simulink model "ukol2"  (R2024b)
settings: Solver=VariableStepAuto  StartTime=0.0  StopTime=40000  RelTol=1e-3
settings Model: Creator=jirka  LastModifiedBy=jirka

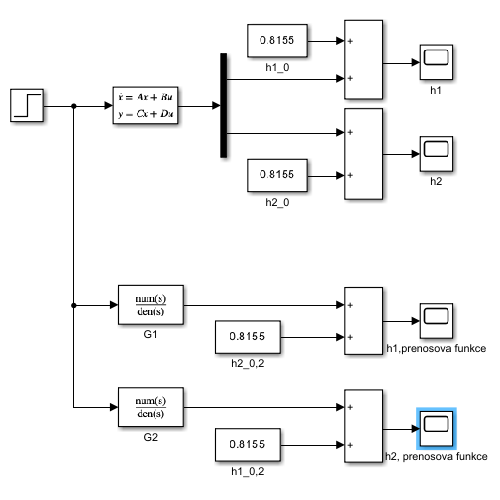
[thumbnail: Simulink's stored preview of the top-level diagram]
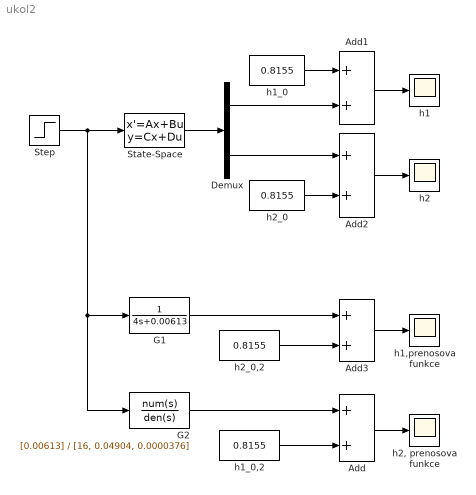
== system ukol2 ==
  Add{,1..3} (4 alike) : Sum
  Demux : Demux  Outputs=2
  G1 : TransferFcn  Denominator=[4, 0.00613]
  G2 : TransferFcn  Numerator=[0.00613]  Denominator=[16, 0.04904, 0.0000376]
  State-Space : StateSpace  A=[-0.00153 0; 0.00153 -0.00153]  B=[0.25; 0]  C=[1 0; 0 1]  D=[0; 0]  InitialCondition=0
  Step : Step  Time=20000  After=0.001  SampleTime=0
  h1 : Scope
  h1,prenosova funkce : Scope
  h1_0 : Constant  Value=0.8155
  h1_0,2 : Constant  Value=0.8155
  h2 : Scope
  "h2, prenosova funkce" : Scope
  h2_0 : Constant  Value=0.8155
  h2_0,2 : Constant  Value=0.8155
  wires:
  Step/1 -> G2/1, G1/1, State-Space/1
  State-Space/1 -> Demux/1
  Demux/2 -> Add2/1
  h1_0/1 -> Add1/1
  h2_0/1 -> Add2/2
  Add1/1 -> h1/1
  Add2/1 -> h2/1
  Demux/1 -> Add1/2
  G2/1 -> Add/1
  h1_0,2/1 -> Add/2
  Add/1 -> "h2, prenosova funkce"/1
  Add3/1 -> h1,prenosova funkce/1
  h2_0,2/1 -> Add3/2
  G1/1 -> Add3/1
